simulink model "RT_ctrl_analyse"  (R2013a)
settings: Solver=ode45  StartTime=0.0  StopTime=10.0  RelTol=1e-3
values from neighbouring files (symbols this model uses):
  fb = 0    [RT_ctrl_analyse_proc.m]
  gain = 1    [RT_ctrl_analyse_proc.m]
  p = sym('p')    [RT_analyse_gui_v1.m]    (also in RT_analyse_gui_v1_BACK.m; RT_analyse_gui_v1a_email_dennis.m; RT_ctrl_analyse_proc.m = [1 1]; RT_lead_lag_uebung.m = -5)
  poles = [-i]    [RT_ctrl_analyse_proc.m]
  z = 8    [RT_ctrl_analyse_proc.m]    (also in RT_lead_lag_uebung.m = -40; regelNormalform_proc.m = [1 p 3])
  zero = []    [RT_ctrl_analyse_proc.m]
settings Model: Creator=mainster  LastModifiedBy=mainster
settings DebuggingCC: SolverPrmCheckMsg=none

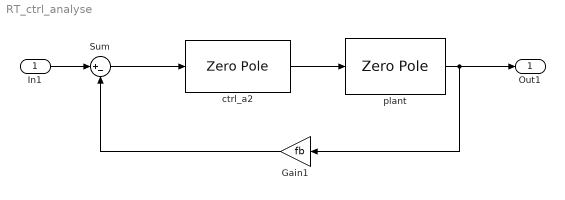
== system RT_ctrl_analyse ==
  In1 : Inport
  Gain1 : Gain  Gain=fb
  Sum : Sum  Inputs=|+-
  ctrl_a2 : ZeroPole  Zeros=zero  Poles=poles  Gain=gain
  plant : ZeroPole  Zeros=[-z]  Poles=[-p]
  Out1 : Outport
  wires:
  In1/1 -> Sum/1
  Gain1/1 -> Sum/2
  Sum/1 -> ctrl_a2/1
  ctrl_a2/1 -> plant/1
  plant/1 -> Out1/1, Gain1/1
